simulink model "Day6Example16and17"  (R2023b)
settings: Solver=VariableStepAuto  StartTime=0.0  StopTime=10.0  RelTol=1e-3
model workspace (MAT data in the model file):
  u = 1.5
settings Model: Creator=ray  LastModifiedBy=ray

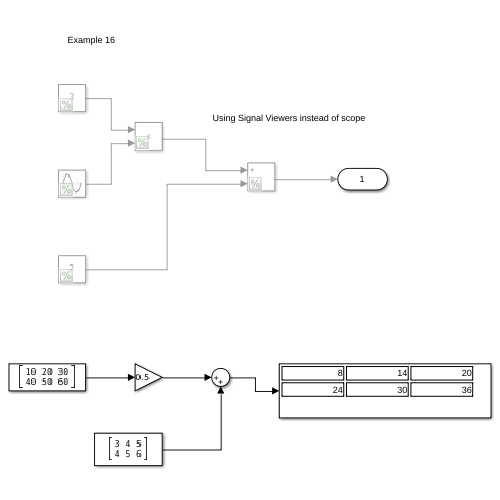
[thumbnail: Simulink's stored preview of the top-level diagram]
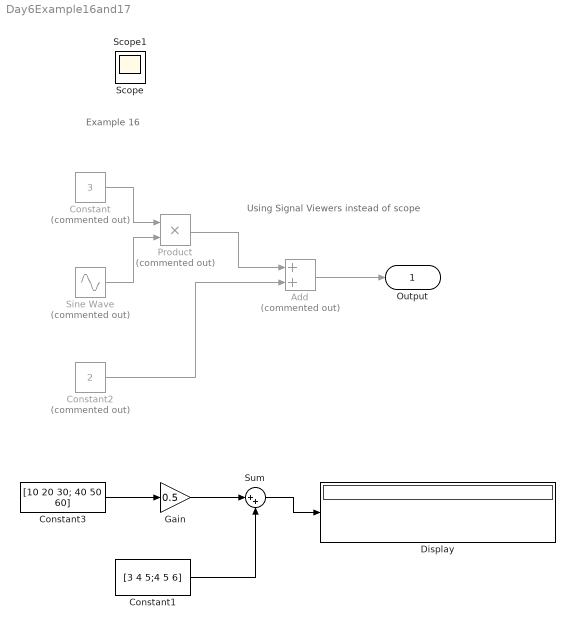
== system Day6Example16and17 ==
  note: Using Signal Viewers instead of scope
  note: Example 16
  Add : Sum  Commented=on
  Constant : Constant  Commented=on  Value=3
  Constant1 : Constant  Value=[3 4 5;4 5 6]
  Constant2 : Constant  Commented=on  Value=2
  Constant3 : Constant  Value=[10 20 30; 40 50 60]
  Display : Display
  Gain : Gain  Gain=0.5
  Product : Product  Commented=on
  Sine Wave : Sin  Commented=on  Amplitude=1.5  SampleTime=0
  Sum : Sum  Inputs=|++
  Output : Outport
  Scope : Scope
  Scope1 : Scope
  wires:
  Constant2/1 -> Add/2
  Add/1 -> Output/1
  Constant/1 -> Product/1
  Sine Wave/1 -> Product/2
  Product/1 -> Add/1
  Constant3/1 -> Gain/1
  Gain/1 -> Sum/1
  Constant1/1 -> Sum/2
  Sum/1 -> Display/1
